simulink model "drone"  (R2023b)
settings: Solver=VariableStepAuto  StartTime=0.0  StopTime=stopTime  RelTol=1e-3
values from neighbouring files (symbols this model uses):
  circle = 0    [oppg3.m]    (also in oppg4.m)
  f_theta = 100/alpha    (= 33.3333333333)    [oppg3.m]
  g = 10    [oppg1.m]    (also in oppg3.m)
  h_ref = 10    [oppg3.m]    (also in oppg4.m)
  k_h_d = 6*2    (= 12)    [oppg3.m]
  k_h_i = 6*2    (= 12)    [oppg3.m]
  k_h_p = 11*2    (= 22)    [oppg3.m]
  k_p_d = 1/20    (= 0.05)    [oppg3.m]
  k_p_p = 1/160    (= 0.00625)    [oppg3.m]
  k_theta_d = 20/alpha    (= 6.66666666667)    [oppg3.m]
  k_theta_p = 100/alpha    (= 33.3333333333)    [oppg3.m]
  M = 2    [oppg1.m]    (also in oppg3.m)
  p_ref = 10    [oppg3.m]    (also in oppg4.m = 100)
settings Model: Creator=hansae  LastModifiedBy=fredr
settings SolverCC: AlgebraicLoopSolver=TrustRegion
settings SFSimCC: CustomCodeUndefinedFunction=UseInterfaceOnly

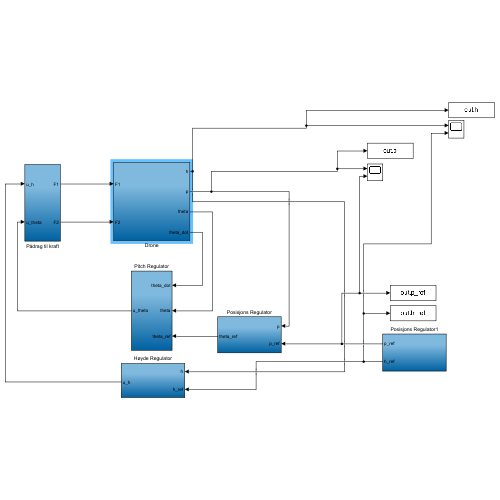
[thumbnail: Simulink's stored preview of the top-level diagram]
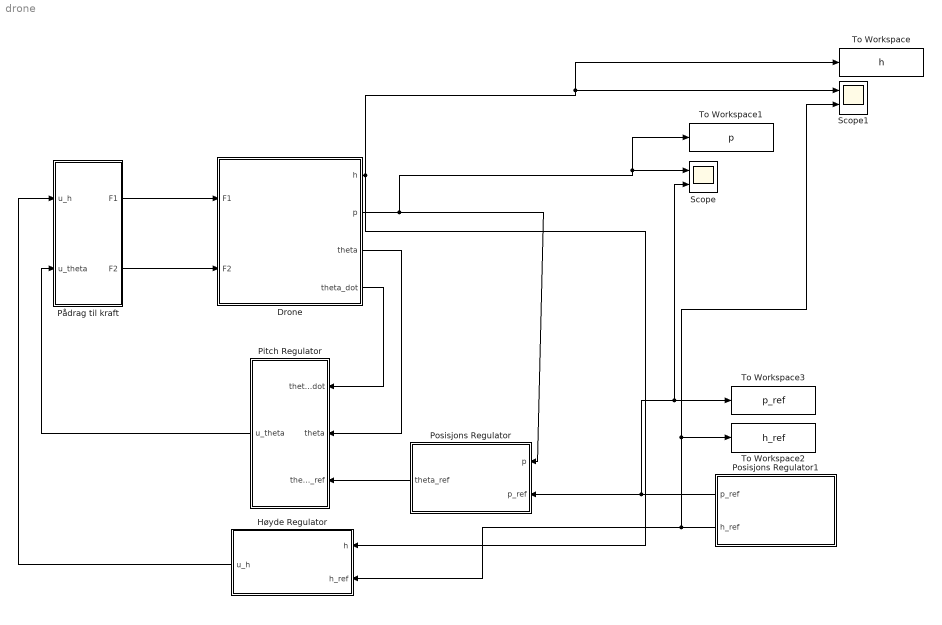
== system drone ==
  Drone : Subsystem
  Høyde Regulator : Subsystem
  Pitch Regulator : Subsystem
  Posisjons Regulator : Subsystem
  Posisjons Regulator1 : Subsystem
  Pådrag til kraft : Subsystem
  Scope : Scope  NumInputPorts=2
  Scope1 : Scope  NumInputPorts=2
  To Workspace : ToWorkspace  VariableName=h  SampleTime=-1
  To Workspace1 : ToWorkspace  VariableName=p  SampleTime=-1
  To Workspace2 : ToWorkspace  VariableName=h_ref  SampleTime=-1
  To Workspace3 : ToWorkspace  VariableName=p_ref  SampleTime=-1
  wires:
  Drone/4(theta_dot) -> Pitch Regulator/1(theta_dot)
  Drone/3(theta) -> Pitch Regulator/2(theta)
  Pitch Regulator/1(u_theta) -> Pådrag til kraft/2(u_theta)
  Posisjons Regulator/1(theta_ref) -> Pitch Regulator/3(theta_ref)
  Pådrag til kraft/1(F1) -> Drone/1(F1)
  Pådrag til kraft/2(F2) -> Drone/2(F2)
  Drone/2(p) -> To Workspace1/1, Scope/1, Posisjons Regulator/1(p)
  Drone/1(h) -> To Workspace/1, Scope1/1, Høyde Regulator/1(h)
  Høyde Regulator/1(u_h) -> Pådrag til kraft/1(u_h)
  Posisjons Regulator1/1(p_ref) -> Scope/2, To Workspace3/1, Posisjons Regulator/2(p_ref)
  Posisjons Regulator1/2(h_ref) -> To Workspace2/1, Scope1/2, Høyde Regulator/2(h_ref)

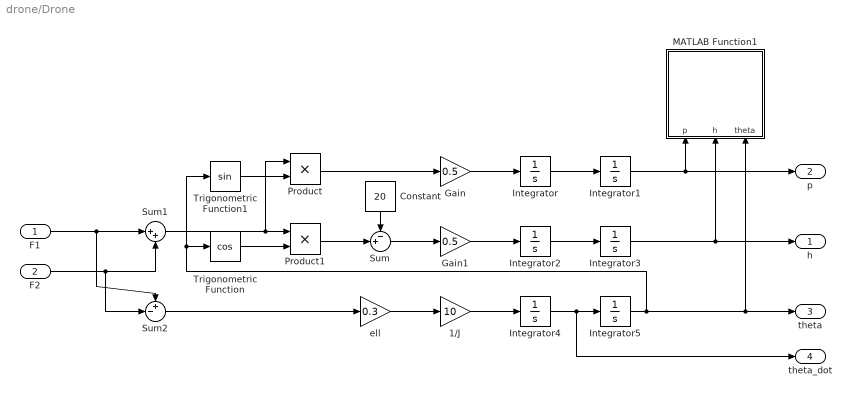
== system drone/Drone ==
  F1 : Inport
  F2 : Inport  Port=2
  1/J : Gain  Gain=10
  Constant : Constant  Value=20
  Gain : Gain  Gain=0.5
  Gain1 : Gain  Gain=0.5
  Integrator{,1..2,4..5} (5 alike) : Integrator
  Integrator3 : Integrator  LimitOutput=on  LowerSaturationLimit=0
  MATLAB Function1 : MATLAB Function  TreatAsAtomicUnit=on  SystemSampleTime=1/30
  Product : Product
  Product1 : Product
  Sum : Sum  Inputs=-+|
  Sum1 : Sum  Inputs=|++
  Sum2 : Sum  Inputs=+-|
  Trigonometric Function : Trigonometry  Operator=cos
  Trigonometric Function1 : Trigonometry
  ell : Gain  Gain=0.3
  h : Outport
  p : Outport  Port=2
  theta : Outport  Port=3
  theta_dot : Outport  Port=4
  wires:
  Integrator3/1 -> h/1, MATLAB Function1/2(h)
  Integrator5/1 -> MATLAB Function1/3(theta), theta/1, Trigonometric Function/1, Trigonometric Function1/1
  Trigonometric Function/1 -> Product1/2
  Integrator4/1 -> theta_dot/1, Integrator5/1
  Product/1 -> Gain/1
  Integrator1/1 -> MATLAB Function1/1(p), p/1
  Sum2/1 -> ell/1
  1/J/1 -> Integrator4/1
  Sum/1 -> Gain1/1
  Trigonometric Function1/1 -> Product/2
  Integrator2/1 -> Integrator3/1
  Integrator/1 -> Integrator1/1
  Gain/1 -> Integrator/1
  F2/1 -> Sum2/2, Sum1/2
  Gain1/1 -> Integrator2/1
  F1/1 -> Sum2/1, Sum1/1
  Sum1/1 -> Product/1, Product1/1
  ell/1 -> 1/J/1
  Constant/1 -> Sum/1
  Product1/1 -> Sum/2

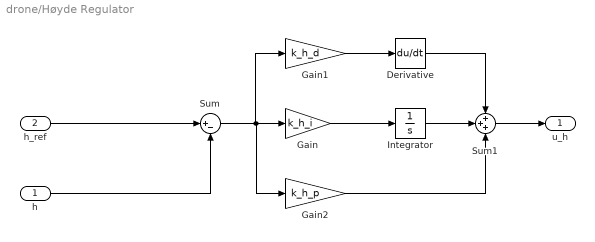
== system drone/Høyde Regulator ==
  h : Inport
  h_ref : Inport  Port=2
  Derivative : Derivative
  Gain : Gain  Gain=k_h_i
  Gain1 : Gain  Gain=k_h_d
  Gain2 : Gain  Gain=k_h_p
  Integrator : Integrator
  Sum : Sum  Inputs=|+-
  Sum1 : Sum  Inputs=+++
  u_h : Outport
  wires:
  Integrator/1 -> Sum1/2
  Derivative/1 -> Sum1/1
  Gain/1 -> Integrator/1
  Sum/1 -> Gain1/1, Gain2/1, Gain/1
  Gain1/1 -> Derivative/1
  Gain2/1 -> Sum1/3
  h_ref/1 -> Sum/1
  h/1 -> Sum/2
  Sum1/1 -> u_h/1

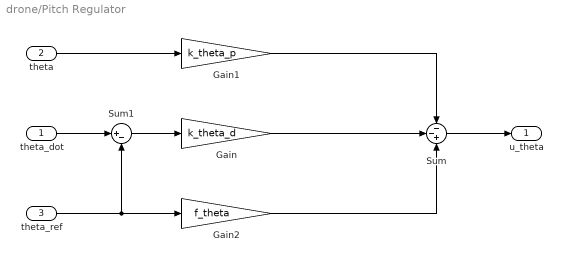
== system drone/Pitch Regulator ==
  theta_dot : Inport
  theta : Inport  Port=2
  theta_ref : Inport  Port=3
  Gain : Gain  Gain=k_theta_d
  Gain1 : Gain  Gain=k_theta_p
  Gain2 : Gain  Gain=f_theta
  Sum : Sum  Inputs=--+
  Sum1 : Sum  Inputs=|+-
  u_theta : Outport
  wires:
  Gain/1 -> Sum/2
  Gain1/1 -> Sum/1
  theta/1 -> Gain1/1
  Gain2/1 -> Sum/3
  theta_ref/1 -> Gain2/1, Sum1/2
  Sum/1 -> u_theta/1
  Sum1/1 -> Gain/1
  theta_dot/1 -> Sum1/1

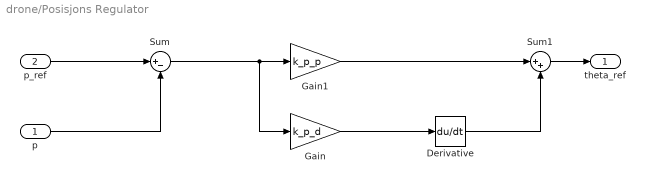
== system drone/Posisjons Regulator ==
  p : Inport
  p_ref : Inport  Port=2
  Derivative : Derivative
  Gain : Gain  Gain=k_p_d
  Gain1 : Gain  Gain=k_p_p
  Sum : Sum  Inputs=|+-
  Sum1 : Sum  Inputs=|++
  theta_ref : Outport
  wires:
  p_ref/1 -> Sum/1
  p/1 -> Sum/2
  Sum/1 -> Gain/1, Gain1/1
  Gain/1 -> Derivative/1
  Sum1/1 -> theta_ref/1
  Derivative/1 -> Sum1/2
  Gain1/1 -> Sum1/1

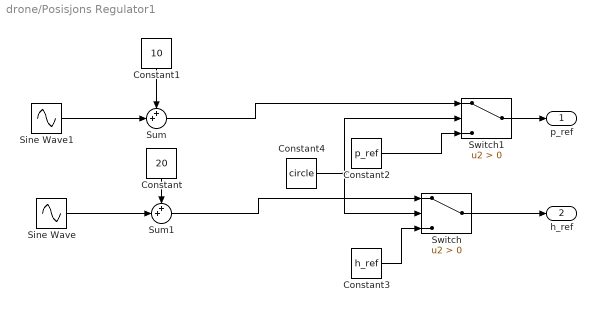
== system drone/Posisjons Regulator1 ==
  Constant : Constant  Value=20
  Constant1 : Constant  Value=10
  Constant2 : Constant  Value=p_ref
  Constant3 : Constant  Value=h_ref
  Constant4 : Constant  Value=circle
  Sine Wave : Sin  Amplitude=5  Frequency=1/4  SampleTime=0
  Sine Wave1 : Sin  Amplitude=5  Frequency=1/4  Phase=pi/2  SampleTime=0
  Sum : Sum  Inputs=++|
  Sum1 : Sum  Inputs=++|
  Switch : Switch  Criteria=u2 > Threshold  SaturateOnIntegerOverflow=off  InputSameDT=off
  Switch1 : Switch  Criteria=u2 > Threshold  SaturateOnIntegerOverflow=off  InputSameDT=off
  p_ref : Outport
  h_ref : Outport  Port=2
  wires:
  Sine Wave/1 -> Sum1/2
  Sine Wave1/1 -> Sum/2
  Constant/1 -> Sum1/1
  Constant1/1 -> Sum/1
  Switch/1 -> h_ref/1
  Constant3/1 -> Switch/3
  Switch1/1 -> p_ref/1
  Constant2/1 -> Switch1/3
  Constant4/1 -> Switch/2, Switch1/2
  Sum1/1 -> Switch/1
  Sum/1 -> Switch1/1

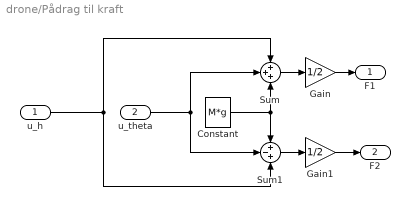
== system drone/Pådrag til kraft ==
  u_h : Inport
  u_theta : Inport  Port=2
  Constant : Constant  Value=M*g
  Gain : Gain  Gain=1/2
  Gain1 : Gain  Gain=1/2
  Sum : Sum  Inputs=+++
  Sum1 : Sum  Inputs=+-+
  F1 : Outport
  F2 : Outport  Port=2
  wires:
  u_theta/1 -> Sum/2, Sum1/2
  Sum/1 -> Gain/1
  Gain/1 -> F1/1
  Sum1/1 -> Gain1/1
  Gain1/1 -> F2/1
  u_h/1 -> Sum/1, Sum1/3
  Constant/1 -> Sum1/1, Sum/3

== matlab function drone/Drone/MATLAB Function1 ==
  settings: updateMethod=DISCRETE
  data: p input; h input; theta input
function plot_drone(p, h, theta)
    % Constants
    N = 40;
    ell = 0.3;

    % Persistent variables
    persistent buffer_p buffer_h writeIdx iter;
    persistent Drone Trace_vector;
    
    % Initialize iteration count
    if isempty(iter)
        iter = 0;
    else
        iter = iter + 1;
    end

    % Buffer Initialization
    if isempty(buffer_p)
        buffer_p = zeros(N, 1);
        buffer_h = zeros(N, 1);
        writeIdx = 1;
    elseif mod(iter, 2) == 0
        buffer_p(writeIdx) = p;
        buffer_h(writeIdx) = h;
        writeIdx = mod(writeIdx, N) + 1;
    end

    % Drone Plot Initialization
    if isempty(Drone)
        Drone = initialize_plot(ell);
    else
        update_drone_position(Drone, p, h, theta);
        drawnow;
    end

    % Trace Vector Initialization
    if isempty(Trace_vector)
        Trace_vector = [hgtransform('parent', gca)];
        for i = 1:N
            Trace_vector = [Trace_vector, hgtransform('parent', gca)];
            plot(0, 0, 'r.', 'markersize', 10, 'Parent', Trace_vector(i));
        end
    elseif mod(iter, 2) == 0
        for i = 1:N
            if ishandle(Trace_vector(i))
                set(Trace_vector(i), 'Matrix', makehgtform('translate', [buffer_p(i), buffer_h(i), 0]));
            end
        end
    end
    
    %% Nested functions
    function Drone = initialize_plot(ell)
        % Setup figure
        figure(1); clf; grid on; hold on; daspect([1, 1, 1]);
        xlim([-2*ell, 2*ell]);
        ylim([-2*ell, 2*ell]);
        xlabel('$p$','interpreter','latex')
        ylabel('$h$','interpreter','latex')

        
        % Draw ground
        yline(-0.47*ell, 'k', 'linewidth', 3);
        
        % Draw drones
        Drone = draw_drone(p, h, ell, 1);
    end

    function update_drone_position(Drone, p, h, theta)
        if ishandle(Drone)
            set(Drone, 'Matrix', makehgtform('translate', [p, h, 0], 'zrotate', -theta));
            xlim([-2*ell, 2*ell] + p);
            ylim([-2*ell, 2*ell] + h);
        end
    end

    function Drone = draw_drone(p,h,ell,opacity)
        % Derived parameters
        w_body = 2*0.27*ell;
        h_body = w_body/2;
        w_prop_body = h_body/2;
        h_prop_body = w_prop_body;
        h_prop_triangle = h_prop_body;
        r_prop = w_body/2;
        dp_feet = 0.4*ell;
        dh_feet = 0.47*ell;
        r_feet = 0.01*ell/0.3;
        r_center = 0.015*ell/0.3;    
        linewidth_narrow = 1;
        linewidth_wide = 2;

        % Drone
        Drone = hgtransform('parent',gca);
        
        % Props
        rectangle('Position',[p+ell-w_prop_body/2,h-h_prop_body,w_prop_body,h_prop_body],'Edgecolor', [0,0,0,opacity],'FaceColor',[1,1,1,opacity],'linewidth',linewidth_narrow,'Parent',Drone);
        rectangle('Position',[p-ell-w_prop_body/2,h-h_prop_body,w_prop_body,h_prop_body],'Edgecolor', [0,0,0,opacity],'FaceColor',[1,1,1,opacity],'linewidth',linewidth_narrow,'Parent',Drone);
        fill([p+ell+w_prop_body/2, p+ell, p+ell-w_prop_body/2, p+ell+w_prop_body/2], [h, h+h_prop_triangle, h, h],'w','FaceAlpha',opacity,'EdgeAlpha',opacity,'linewidth',linewidth_narrow,'Parent',Drone);
        fill([p-ell+w_prop_body/2, p-ell, p-ell-w_prop_body/2, p-ell+w_prop_body/2], [h, h+h_prop_triangle, h, h],'w','FaceAlpha',opacity,'EdgeAlpha',opacity,'linewidth',linewidth_narrow,'Parent',Drone);
        line([p+ell-r_prop, p+ell+r_prop], [h+2*h_prop_triangle/4, h+2*h_prop_triangle/4],'linewidth',linewidth_narrow,'color',[0,0,0,opacity],'Parent',Drone);
        line([p-ell-r_prop, p-ell+r_prop], [h+2*h_prop_triangle/4, h+2*h_prop_triangle/4],'linewidth',linewidth_narrow,'color',[0,0,0,opacity],'Parent',Drone);
        
        % Feet
        alpha = 0.28; % Hack to fix feet being visible through body when transparent
        line([p+alpha*dp_feet,p+dp_feet],[h-alpha*dh_feet,h-dh_feet],'linewidth',linewidth_narrow,'color',[0,0,0,opacity],'Parent',Drone);
        line([p-alpha*dp_feet,p-dp_feet],[h-alpha*dh_feet,h-dh_feet],'linewidth',linewidth_narrow,'color',[0,0,0,opacity],'Parent',Drone);
        rectangle('Position',[p+dp_feet-r_feet/2,h-dh_feet-r_feet/2,r_feet,r_feet],'Curvature',1,'Edgecolor', [0,0,0,opacity],'FaceColor',[0,0,0,opacity],'linewidth',linewidth_narrow,'Parent',Drone);
        rectangle('Position',[p-dp_feet-r_feet/2,h-dh_feet-r_feet/2,r_feet,r_feet],'Curvature',1,'Edgecolor', [0,0,0,opacity],'FaceColor',[0,0,0,opacity],'linewidth',linewidth_narrow,'Parent',Drone);
        
        % Arms
        line([p+w_body/2,p+ell+w_prop_body/2],[0,0],'linewidth',linewidth_wide,'color',[0,0,0,opacity],'Parent',Drone);
        line([p-w_body/2,p-ell-w_prop_body/2],[0,0],'linewidth',linewidth_wide,'color',[0,0,0,opacity],'Parent',Drone);
        
        % Body
        rectangle('Position',[p-w_body/2,h-h_body/2,w_body,h_body],'Edgecolor', [0,0,0,opacity],'FaceColor',[1,1,1,opacity],'linewidth',linewidth_narrow,'Parent',Drone);
        rectangle('Position',[p-r_center/2,h-r_center/2,r_center,r_center],'Curvature',1,'Edgecolor', [0,0,0,opacity],'FaceColor',[0,0,0,opacity],'linewidth',linewidth_narrow,'Parent',Drone);
    end
end
